simulink model "StaticFeedback"  (R2021a)
settings: Solver=ode113  StartTime=0.0  StopTime=10.0  RelTol=1e-3
values from neighbouring files (symbols this model uses):
  A = [0 1 0 0; (m+M)*g/(M*L) 0 0 0; 0 0 0 1; (-m*g)/M 0 0 0]    [StateSpaceREP.m]
  B = [0; -1/M*L; 0; 1/M]    [StateSpaceREP.m]
  C_block = eye(4)    [StateSpaceREP.m]
  D_block = zeros(4,1)    [StateSpaceREP.m]
  F = -acker(A,B,desiredEigen)    [StateSpaceREP.m]
settings Model: Creator=pbmellache2020  LastModifiedBy=pbmellache2020
settings DataIOCC: ReturnWorkspaceOutputs=off

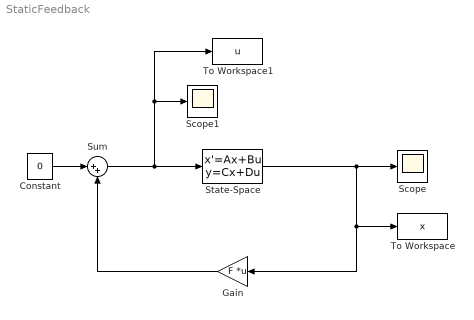
== system StaticFeedback ==
  Constant : Constant  Value=0
  Gain : Gain  Gain=F  Multiplication=Matrix(K*u)
  Scope : Scope
  Scope1 : Scope
  State-Space : StateSpace  A=A  B=B  C=C_block  D=D_block  InitialCondition=[0.1 0 0.1 0]
  Sum : Sum  Inputs=|++
  To Workspace : ToWorkspace  VariableName=x  SampleTime=-1
  To Workspace1 : ToWorkspace  VariableName=u  SampleTime=-1
  wires:
  Sum/1 -> To Workspace1/1, Scope1/1, State-Space/1
  State-Space/1 -> Scope/1, To Workspace/1, Gain/1
  Gain/1 -> Sum/2
  Constant/1 -> Sum/1
